simulink library "simulink"  (Simulink 6.0)
settings: Solver=ode45  SolverMode=SingleTasking  StartTime=0.0  StopTime=10.0  RelTol=1e-3
PostLoadFcn:
  | setsysloc(bdroot)
undefined symbols (not defined in the file or in its folder): DiscIntNeverNeededParam, getdatatypespecs, NumBits1, NumBits2, sfunxy, sigbuilder_block, slcm, Slope1, Slope2
libraries: simulink x82, eml_lib x1
(part 5 of 5)

== system simulink/Lookup Tables/Sine/Handle Quarter Symetery Sine ==
  Raw Angle : Inport  LatchInput=off
  Output From Lookup Table : Inport  Port=2  LatchInput=off
  Amp50 : Sum  Inputs=+-  OutDataType=uint(8)  OutScaling=1  LockScale=on
  CastU16En16 : DataTypeConversion  OutDataTypeMode=Specify via dialog  OutDataType=ufix(16)  OutScaling=2^-16  LockScale=on
  LTEp25 : RelationalOperator  Operator=<=  LogicOutDataTypeMode=Specify via dialog  ZeroCross=off
  LTEp50 : RelationalOperator  Operator=<=  LogicOutDataTypeMode=Specify via dialog  ZeroCross=off
  Negate : simulink/Math Operations/Unary Minus  DoSatur=off
  Point25 : Constant  Value=0.25  OutDataTypeMode=Specify via dialog  OutDataType=ufix(16)  OutScaling=2^-16
  Point50 : Constant  Value=0.5  OutDataTypeMode=Specify via dialog  OutDataType=ufix(16)  OutScaling=2^-16
  QuadHandle1 : Switch  Criteria=u2 ~= 0  ZeroCross=off
  QuadHandle2 : Switch  Criteria=u2 ~= 0  ZeroCross=off
  SignCorrected : Switch  Threshold=1  ZeroCross=off
  p50mA : Sum  Inputs=+-  OutDataType=uint(8)  OutScaling=1  LockScale=on
  Sine : Outport
  Input To Lookup Table : Outport  Port=2
  wires:
  Raw Angle/1 -> CastU16En16/1
  LTEp50/1 -> QuadHandle1/2, SignCorrected/2
  QuadHandle1/1 -> LTEp25/1, QuadHandle2/1, p50mA/2
  Point25/1 -> LTEp25/2
  LTEp25/1 -> QuadHandle2/2
  QuadHandle2/1 -> Input To Lookup Table/1
  CastU16En16/1 -> LTEp50/1, QuadHandle1/1, Amp50/1
  Output From Lookup Table/1 -> Negate/1, SignCorrected/1
  SignCorrected/1 -> Sine/1
  Amp50/1 -> QuadHandle1/3
  Negate/1 -> SignCorrected/3
  p50mA/1 -> QuadHandle2/3
  Point50/1 -> LTEp50/2, Amp50/2, p50mA/1

== system simulink/Model Verification/Check Input  Resolution/fixed ==
  u : Inport  LatchInput=off
  resolution : Inport  Port=2  LatchInput=off
  fold : Logic  Operator=OR  Inputs=1
  relop : RelationalOperator  Operator===  InputSameDT=on
  out : Outport
  wires:
  u/1 -> relop/1
  resolution/1 -> relop/2
  relop/1 -> fold/1
  fold/1 -> out/1

== system simulink/Model Verification/Check Input  Resolution/steps ==
  u : Inport  LatchInput=off
  resolution : Inport  Port=2  LatchInput=off
  relop : RelationalOperator  Operator=<=  InputSameDT=on
  rem : Math  Operator=mod  SaturateOnIntegerOverflow=on
  tol : Constant  Value=10e-3
  out : Outport
  wires:
  u/1 -> rem/1
  resolution/1 -> rem/2
  rem/1 -> relop/1
  tol/1 -> relop/2
  relop/1 -> out/1

== system simulink/Model-Wide Utilities/Block Support Table/EmptySubsystem ==

== system simulink/Model-Wide Utilities/DocBlock/EmptySubsystem ==

== system simulink/Model-Wide Utilities/Model Info/EmptySubsystem ==

== system simulink/Model-Wide Utilities/Timed-Based Linearization/Triggered Linearization ==
  Trigger : TriggerPort
  S-Function : S-Function  FunctionName=sfunlin  Parameters=name_,SampleTime
